simulink model "case7"  (R2024b)
settings: Solver=FixedStepAuto  StartTime=0  StopTime=1  FixedStep=1e-7  RelTol=1e-3
values from neighbouring files (symbols this model uses):
  SG_D_1_D = 0.01056    [IEEE9_case_parameters.m]    (also in case1_parameters.m; case2_parameters.m; case3_parameters.m; case4_parameters.m)
  SG_D_1_EnableSaturation = 0    [IEEE9_case_parameters.m]    (also in case1_parameters.m; case2_parameters.m; case3_parameters.m; case4_parameters.m)
  SG_D_1_f0 = 60    [IEEE9_case_parameters.m]    (also in case1_parameters.m; case2_parameters.m; case3_parameters.m; case4_parameters.m)
  SG_D_1_H = 7.5    [IEEE9_case_parameters.m]    (also in case1_parameters.m; case2_parameters.m; case3_parameters.m; case4_parameters.m)
  SG_D_1_K_A = 20    [IEEE9_case_parameters.m]    (also in case1_parameters.m; case2_parameters.m; case3_parameters.m; case4_parameters.m)
  SG_D_1_K_E = 1.000000e+1    (= 10)    [IEEE9_case_parameters.m]    (also in case1_parameters.m; case2_parameters.m; case3_parameters.m; case4_parameters.m)
  SG_D_1_K_F = 2.363    [IEEE9_case_parameters.m]    (also in case1_parameters.m; case2_parameters.m; case3_parameters.m; case4_parameters.m)
  SG_D_1_K_s = 0.5    [IEEE9_case_parameters.m]    (also in case1_parameters.m = 5; case2_parameters.m = 5; case3_parameters.m = 5; case4_parameters.m = 5)
  SG_D_1_R_a = 0.001088    [IEEE9_case_parameters.m]    (also in case1_parameters.m; case2_parameters.m; case3_parameters.m; case4_parameters.m)
  SG_D_1_S_A = 1    [IEEE9_case_parameters.m]    (also in case1_parameters.m; case2_parameters.m; case3_parameters.m; case4_parameters.m)
  SG_D_1_S_B = 0.103    [IEEE9_case_parameters.m]    (also in case1_parameters.m; case2_parameters.m; case3_parameters.m; case4_parameters.m)
  SG_D_1_S_N = 10.659857    [IEEE9_case_parameters.m]    (also in case1_parameters.m; case2_parameters.m; case3_parameters.m; case4_parameters.m)
  SG_D_1_SpeedPara = 200    [IEEE9_case_parameters.m]    (also in case1_parameters.m; case2_parameters.m; case3_parameters.m; case4_parameters.m)
  SG_D_1_T_0 = 0.720173    [IEEE9_case_parameters.m]    (also in case1_parameters.m = 0.755522; case2_parameters.m = 0.808931; case3_parameters.m = 0.869402; case4_parameters.m = 0.729316)
  SG_D_1_T_1 = 0.3    [IEEE9_case_parameters.m]    (also in case1_parameters.m; case2_parameters.m; case3_parameters.m; case4_parameters.m)
  SG_D_1_T_2 = 0.05    [IEEE9_case_parameters.m]    (also in case1_parameters.m; case2_parameters.m; case3_parameters.m; case4_parameters.m)
  SG_D_1_T_3 = 0.02    [IEEE9_case_parameters.m]    (also in case1_parameters.m; case2_parameters.m; case3_parameters.m; case4_parameters.m)
  SG_D_1_T_4 = 0.005    [IEEE9_case_parameters.m]    (also in case1_parameters.m; case2_parameters.m; case3_parameters.m; case4_parameters.m)
  SG_D_1_T_A = 0.02    [IEEE9_case_parameters.m]    (also in case1_parameters.m; case2_parameters.m; case3_parameters.m; case4_parameters.m)
  SG_D_1_T_dd = 8.000000e+0    (= 8)    [IEEE9_case_parameters.m]    (also in case1_parameters.m; case2_parameters.m; case3_parameters.m; case4_parameters.m)
  SG_D_1_T_ddd = 0.04    [IEEE9_case_parameters.m]    (also in case1_parameters.m; case2_parameters.m; case3_parameters.m; case4_parameters.m)
  SG_D_1_T_E = 0.314    [IEEE9_case_parameters.m]    (also in case1_parameters.m; case2_parameters.m; case3_parameters.m; case4_parameters.m)
  SG_D_1_T_F = 0.35    [IEEE9_case_parameters.m]    (also in case1_parameters.m; case2_parameters.m; case3_parameters.m; case4_parameters.m)
  SG_D_1_T_qd = 0.8    [IEEE9_case_parameters.m]    (also in case1_parameters.m; case2_parameters.m; case3_parameters.m; case4_parameters.m)
  SG_D_1_T_qdd = 0.02    [IEEE9_case_parameters.m]    (also in case1_parameters.m; case2_parameters.m; case3_parameters.m; case4_parameters.m)
  SG_D_1_T_speed = 0.1    [IEEE9_case_parameters.m]    (also in case1_parameters.m = 200; case2_parameters.m = 200; case3_parameters.m = 200; case4_parameters.m = 200)
  SG_D_1_T_w = 0.5    [IEEE9_case_parameters.m]    (also in case1_parameters.m; case2_parameters.m; case3_parameters.m; case4_parameters.m)
  SG_D_1_V_ref = 1.990276    [IEEE9_case_parameters.m]    (also in case1_parameters.m = 2.042296; case2_parameters.m = 2.051388; case3_parameters.m = 2.089584; case4_parameters.m = 2.01845)
  SG_D_1_w_ref = 376.991118    [IEEE9_case_parameters.m]    (also in case1_parameters.m; case2_parameters.m; case3_parameters.m; case4_parameters.m)
  SG_D_1_wb = 6.000000e+1    (= 60)    [IEEE9_case_parameters.m]    (also in case1_parameters.m; case2_parameters.m; case3_parameters.m; case4_parameters.m)
  SG_D_1_x_d = 1.9    [IEEE9_case_parameters.m]    (also in case1_parameters.m; case2_parameters.m; case3_parameters.m; case4_parameters.m)
  SG_D_1_x_dd = 0.302    [IEEE9_case_parameters.m]    (also in case1_parameters.m; case2_parameters.m; case3_parameters.m; case4_parameters.m)
  SG_D_1_x_ddd = 0.204    [IEEE9_case_parameters.m]    (also in case1_parameters.m; case2_parameters.m; case3_parameters.m; case4_parameters.m)
  SG_D_1_x_l = 0.05    [IEEE9_case_parameters.m]    (also in case1_parameters.m; case2_parameters.m; case3_parameters.m; case4_parameters.m)
  SG_D_1_x_q = 1.3    [IEEE9_case_parameters.m]    (also in case1_parameters.m; case2_parameters.m; case3_parameters.m; case4_parameters.m)
  SG_D_1_x_qd = 0.5    [IEEE9_case_parameters.m]    (also in case1_parameters.m; case2_parameters.m; case3_parameters.m; case4_parameters.m)
  SG_D_1_x_qdd = 0.3    [IEEE9_case_parameters.m]    (also in case1_parameters.m; case2_parameters.m; case3_parameters.m; case4_parameters.m)
  SG_D_2_D = 0.02    [IEEE9_case_parameters.m]    (also in case1_parameters.m; case2_parameters.m; case3_parameters.m; case4_parameters.m)
  SG_D_2_EnableSaturation = 0    [IEEE9_case_parameters.m]    (also in case1_parameters.m; case2_parameters.m; case3_parameters.m; case4_parameters.m)
  SG_D_2_f0 = 60    [IEEE9_case_parameters.m]    (also in case1_parameters.m; case2_parameters.m; case3_parameters.m; case4_parameters.m)
  SG_D_2_H = 8.000000e+0    (= 8)    [IEEE9_case_parameters.m]    (also in case1_parameters.m; case2_parameters.m; case3_parameters.m; case4_parameters.m)
  SG_D_2_K_A = 20    [IEEE9_case_parameters.m]    (also in case1_parameters.m; case2_parameters.m; case3_parameters.m; case4_parameters.m)
  SG_D_2_K_E = 1.000000e+1    (= 10)    [IEEE9_case_parameters.m]    (also in case1_parameters.m; case2_parameters.m; case3_parameters.m; case4_parameters.m)
  SG_D_2_K_F = 2.363    [IEEE9_case_parameters.m]    (also in case1_parameters.m; case2_parameters.m; case3_parameters.m; case4_parameters.m)
  SG_D_2_K_s = 0.5    [IEEE9_case_parameters.m]    (also in case1_parameters.m = 4; case2_parameters.m = 4; case3_parameters.m = 4; case4_parameters.m = 4)
  SG_D_2_R_a = 0.001088    [IEEE9_case_parameters.m]    (also in case1_parameters.m; case2_parameters.m; case3_parameters.m; case4_parameters.m)
  SG_D_2_S_A = 1    [IEEE9_case_parameters.m]    (also in case1_parameters.m; case2_parameters.m; case3_parameters.m; case4_parameters.m)
  SG_D_2_S_B = 0.103    [IEEE9_case_parameters.m]    (also in case1_parameters.m; case2_parameters.m; case3_parameters.m; case4_parameters.m)
  SG_D_2_S_N = 10.659857    [IEEE9_case_parameters.m]    (also in case1_parameters.m; case2_parameters.m; case3_parameters.m; case4_parameters.m)
  SG_D_2_SpeedPara = 200    [IEEE9_case_parameters.m]    (also in case1_parameters.m; case2_parameters.m; case3_parameters.m; case4_parameters.m)
  SG_D_2_T_0 = 1.632913    [IEEE9_case_parameters.m]    (also in case1_parameters.m = 1.632925; case2_parameters.m = 1.632915; case3_parameters.m = 1.632914; case4_parameters.m = 1.632927)
  SG_D_2_T_1 = 0.2    [IEEE9_case_parameters.m]    (also in case1_parameters.m; case2_parameters.m; case3_parameters.m; case4_parameters.m)
  SG_D_2_T_2 = 0.05    [IEEE9_case_parameters.m]    (also in case1_parameters.m; case2_parameters.m; case3_parameters.m; case4_parameters.m)
  SG_D_2_T_3 = 0.02    [IEEE9_case_parameters.m]    (also in case1_parameters.m; case2_parameters.m; case3_parameters.m; case4_parameters.m)
  SG_D_2_T_4 = 0.005    [IEEE9_case_parameters.m]    (also in case1_parameters.m; case2_parameters.m; case3_parameters.m; case4_parameters.m)
  SG_D_2_T_A = 0.02    [IEEE9_case_parameters.m]    (also in case1_parameters.m; case2_parameters.m; case3_parameters.m; case4_parameters.m)
  SG_D_2_T_dd = 7.9    [IEEE9_case_parameters.m]    (also in case1_parameters.m; case2_parameters.m; case3_parameters.m; case4_parameters.m)
  SG_D_2_T_ddd = 0.04    [IEEE9_case_parameters.m]    (also in case1_parameters.m; case2_parameters.m; case3_parameters.m; case4_parameters.m)
  SG_D_2_T_E = 0.314    [IEEE9_case_parameters.m]    (also in case1_parameters.m; case2_parameters.m; case3_parameters.m; case4_parameters.m)
  SG_D_2_T_F = 0.35    [IEEE9_case_parameters.m]    (also in case1_parameters.m; case2_parameters.m; case3_parameters.m; case4_parameters.m)
  SG_D_2_T_qd = 0.8    [IEEE9_case_parameters.m]    (also in case1_parameters.m; case2_parameters.m; case3_parameters.m; case4_parameters.m)
  SG_D_2_T_qdd = 0.015    [IEEE9_case_parameters.m]    (also in case1_parameters.m; case2_parameters.m; case3_parameters.m; case4_parameters.m)
  SG_D_2_T_speed = 0.1    [IEEE9_case_parameters.m]    (also in case1_parameters.m = 150; case2_parameters.m = 150; case3_parameters.m = 150; case4_parameters.m = 150)
  SG_D_2_T_w = 0.35    [IEEE9_case_parameters.m]    (also in case1_parameters.m; case2_parameters.m; case3_parameters.m; case4_parameters.m)
  SG_D_2_V_ref = 2.58547    [IEEE9_case_parameters.m]    (also in case1_parameters.m = 2.597896; case2_parameters.m = 2.587136; case3_parameters.m = 2.586042; case4_parameters.m = 2.599679)
  SG_D_2_w_ref = 376.991118    [IEEE9_case_parameters.m]    (also in case1_parameters.m; case2_parameters.m; case3_parameters.m; case4_parameters.m)
  SG_D_2_wb = 6.000000e+1    (= 60)    [IEEE9_case_parameters.m]    (also in case1_parameters.m; case2_parameters.m; case3_parameters.m; case4_parameters.m)
  SG_D_2_x_d = 1.8    [IEEE9_case_parameters.m]    (also in case1_parameters.m; case2_parameters.m; case3_parameters.m; case4_parameters.m)
  SG_D_2_x_dd = 0.302    [IEEE9_case_parameters.m]    (also in case1_parameters.m; case2_parameters.m; case3_parameters.m; case4_parameters.m)
  SG_D_2_x_ddd = 0.204    [IEEE9_case_parameters.m]    (also in case1_parameters.m; case2_parameters.m; case3_parameters.m; case4_parameters.m)
  SG_D_2_x_l = 0.05    [IEEE9_case_parameters.m]    (also in case1_parameters.m; case2_parameters.m; case3_parameters.m; case4_parameters.m)
  SG_D_2_x_q = 1.25    [IEEE9_case_parameters.m]    (also in case1_parameters.m; case2_parameters.m; case3_parameters.m; case4_parameters.m)
  SG_D_2_x_qd = 0.5    [IEEE9_case_parameters.m]    (also in case1_parameters.m; case2_parameters.m; case3_parameters.m; case4_parameters.m)
  SG_D_2_x_qdd = 0.3    [IEEE9_case_parameters.m]    (also in case1_parameters.m; case2_parameters.m; case3_parameters.m; case4_parameters.m)
  SG_D_3_D = 0.02    [IEEE9_case_parameters.m]    (also in case1_parameters.m; case2_parameters.m; case3_parameters.m; case4_parameters.m)
  SG_D_3_EnableSaturation = 0    [IEEE9_case_parameters.m]    (also in case1_parameters.m; case2_parameters.m; case3_parameters.m; case4_parameters.m)
  SG_D_3_f0 = 60    [IEEE9_case_parameters.m]    (also in case1_parameters.m; case2_parameters.m; case3_parameters.m; case4_parameters.m)
  SG_D_3_H = 7.7    [IEEE9_case_parameters.m]    (also in case1_parameters.m; case2_parameters.m; case3_parameters.m; case4_parameters.m)
  SG_D_3_K_A = 20    [IEEE9_case_parameters.m]    (also in case1_parameters.m; case2_parameters.m; case3_parameters.m; case4_parameters.m)
  SG_D_3_K_E = 1.000000e+1    (= 10)    [IEEE9_case_parameters.m]    (also in case1_parameters.m; case2_parameters.m; case3_parameters.m; case4_parameters.m)
  SG_D_3_K_F = 2.363    [IEEE9_case_parameters.m]    (also in case1_parameters.m; case2_parameters.m; case3_parameters.m; case4_parameters.m)
  SG_D_3_K_s = 0.2    [IEEE9_case_parameters.m]    (also in case1_parameters.m = 2; case2_parameters.m = 2; case3_parameters.m = 2; case4_parameters.m = 2)
  SG_D_3_R_a = 0.001088    [IEEE9_case_parameters.m]    (also in case1_parameters.m; case2_parameters.m; case3_parameters.m; case4_parameters.m)
  SG_D_3_S_A = 1    [IEEE9_case_parameters.m]    (also in case1_parameters.m; case2_parameters.m; case3_parameters.m; case4_parameters.m)
  SG_D_3_S_B = 0.103    [IEEE9_case_parameters.m]    (also in case1_parameters.m; case2_parameters.m; case3_parameters.m; case4_parameters.m)
  SG_D_3_S_N = 10.659857    [IEEE9_case_parameters.m]    (also in case1_parameters.m; case2_parameters.m; case3_parameters.m; case4_parameters.m)
  SG_D_3_SpeedPara = 200    [IEEE9_case_parameters.m]    (also in case1_parameters.m; case2_parameters.m; case3_parameters.m; case4_parameters.m)
  SG_D_3_T_0 = 0.850788    [IEEE9_case_parameters.m]    (also in case1_parameters.m = 0.850786; case2_parameters.m = 0.850787; case3_parameters.m; case4_parameters.m = 0.850786)
  SG_D_3_T_1 = 0.2    [IEEE9_case_parameters.m]    (also in case1_parameters.m; case2_parameters.m; case3_parameters.m; case4_parameters.m)
  SG_D_3_T_2 = 0.05    [IEEE9_case_parameters.m]    (also in case1_parameters.m; case2_parameters.m; case3_parameters.m; case4_parameters.m)
  SG_D_3_T_3 = 0.02    [IEEE9_case_parameters.m]    (also in case1_parameters.m; case2_parameters.m; case3_parameters.m; case4_parameters.m)
  SG_D_3_T_4 = 0.005    [IEEE9_case_parameters.m]    (also in case1_parameters.m; case2_parameters.m; case3_parameters.m; case4_parameters.m)
  SG_D_3_T_A = 0.02    [IEEE9_case_parameters.m]    (also in case1_parameters.m; case2_parameters.m; case3_parameters.m; case4_parameters.m)
  SG_D_3_T_dd = 8.1    [IEEE9_case_parameters.m]    (also in case1_parameters.m; case2_parameters.m; case3_parameters.m; case4_parameters.m)
  SG_D_3_T_ddd = 0.04    [IEEE9_case_parameters.m]    (also in case1_parameters.m; case2_parameters.m; case3_parameters.m; case4_parameters.m)
  SG_D_3_T_E = 0.314    [IEEE9_case_parameters.m]    (also in case1_parameters.m; case2_parameters.m; case3_parameters.m; case4_parameters.m)
  SG_D_3_T_F = 0.35    [IEEE9_case_parameters.m]    (also in case1_parameters.m; case2_parameters.m; case3_parameters.m; case4_parameters.m)
  SG_D_3_T_qd = 0.8    [IEEE9_case_parameters.m]    (also in case1_parameters.m; case2_parameters.m; case3_parameters.m; case4_parameters.m)
  SG_D_3_T_qdd = 0.015    [IEEE9_case_parameters.m]    (also in case1_parameters.m; case2_parameters.m; case3_parameters.m; case4_parameters.m)
  SG_D_3_T_speed = 0.1    [IEEE9_case_parameters.m]    (also in case1_parameters.m = 180; case2_parameters.m = 180; case3_parameters.m = 180; case4_parameters.m = 180)
  SG_D_3_T_w = 0.4    [IEEE9_case_parameters.m]    (also in case1_parameters.m; case2_parameters.m; case3_parameters.m; case4_parameters.m)
  SG_D_3_V_ref = 1.892727    [IEEE9_case_parameters.m]    (also in case1_parameters.m = 1.906439; case2_parameters.m = 1.895535; case3_parameters.m = 1.892105; case4_parameters.m = 1.906598)
  SG_D_3_w_ref = 376.991118    [IEEE9_case_parameters.m]    (also in case1_parameters.m; case2_parameters.m; case3_parameters.m; case4_parameters.m)
  SG_D_3_wb = 6.000000e+1    (= 60)    [IEEE9_case_parameters.m]    (also in case1_parameters.m; case2_parameters.m; case3_parameters.m; case4_parameters.m)
  SG_D_3_x_d = 1.85    [IEEE9_case_parameters.m]    (also in case1_parameters.m; case2_parameters.m; case3_parameters.m; case4_parameters.m)
  SG_D_3_x_dd = 0.302    [IEEE9_case_parameters.m]    (also in case1_parameters.m; case2_parameters.m; case3_parameters.m; case4_parameters.m)
  SG_D_3_x_ddd = 0.204    [IEEE9_case_parameters.m]    (also in case1_parameters.m; case2_parameters.m; case3_parameters.m; case4_parameters.m)
  SG_D_3_x_l = 0.05    [IEEE9_case_parameters.m]    (also in case1_parameters.m; case2_parameters.m; case3_parameters.m; case4_parameters.m)
  SG_D_3_x_q = 1.2    [IEEE9_case_parameters.m]    (also in case1_parameters.m; case2_parameters.m; case3_parameters.m; case4_parameters.m)
  SG_D_3_x_qd = 0.5    [IEEE9_case_parameters.m]    (also in case1_parameters.m; case2_parameters.m; case3_parameters.m; case4_parameters.m)
  SG_D_3_x_qdd = 0.3    [IEEE9_case_parameters.m]    (also in case1_parameters.m; case2_parameters.m; case3_parameters.m; case4_parameters.m)
(part 6 of 12)

== system case7/SG_D_1/d_psi_kq_SG_D_1_block ==
  note: d_psi_kq_SG_D_1 in case7
      | $-\frac{\psi _{\mathrm{gq},\mathrm{SG},D,1}+\psi _{\mathrm{kq},\mathrm{SG},D,1}+\frac{\left(x_{l}-x_{\mathrm{qd}}\right)\,\left(\psi _{q,\mathrm{SG},D,1}+\frac{\psi _{\mathrm{gq},\mathrm{SG},D,1}\,\left(x_{l}-x_{\mathrm{qdd}}\right)}{x_{l}-x_{\mathrm{qd}}}+\frac{\psi _{\mathrm{kq},\mathrm{SG},D,1}\,\left(x_{\mathrm{qd}}-x_{\mathrm{qdd}}\right)}{x_{l}-x_{\mathrm{qd}}}\right)}{x_{\mathrm{qdd}}}}{T_{\mathrm{qdd}}}$
      | Automatically generated on 2025-10-31 19:23:24 .
  State_psi_gq_SG_D_1_141c0 : Inport
  State_psi_kq_SG_D_1_73ccc : Inport  Port=2
  State_psi_gq_SG_D_1_32f50 : Inport  Port=3
  State_psi_kq_SG_D_1_9c021 : Inport  Port=4
  State_psi_q_SG_D_1_95dfc : Inport  Port=5
  Add_4d238 : Sum
  Add_52c21 : Sum
  Add_5b3bd : Sum
  Add_78e01 : Sum
  Add_7e5bc : Sum
  Add_abf74 : Sum
  Constant_-1_7f4f9 : Constant  Value=-1
  Constant_-1_8033d : Constant  Value=-1
  Constant_-1_939f1 : Constant  Value=-1
  Constant_-1_ca431 : Constant  Value=-1
  Constant_-1_cc594 : Constant  Value=-1
  Constant_T_qdd_ef478 : Constant  Value=T_qdd
  Constant_x_l_00713 : Constant  Value=x_l
  Constant_x_l_01d91 : Constant  Value=x_l
  Constant_x_l_4eb42 : Constant  Value=x_l
  Constant_x_l_702c1 : Constant  Value=x_l
  Constant_x_qd_06ea1 : Constant  Value=x_qd
  Constant_x_qd_55376 : Constant  Value=x_qd
  Constant_x_qd_bc9ff : Constant  Value=x_qd
  Constant_x_qd_cd86c : Constant  Value=x_qd
  Constant_x_qdd_04518 : Constant  Value=x_qdd
  Constant_x_qdd_b13f8 : Constant  Value=x_qdd
  Constant_x_qdd_e31b1 : Constant  Value=x_qdd
  Divide_172d7 : Product  Inputs=*/
  Divide_318ea : Product  Inputs=*/
  Divide_dd02d : Product  Inputs=*/
  Divide_ff5c9 : Product  Inputs=*/
  Product_49e9a : Product
  Product_575bc : Product
  Product_595ac : Product
  Product_801da : Product
  Product_92b80 : Product
  Product_9c9eb : Product
  Product_d5d1d : Product
  Product_e2544 : Product
  Subtract_41446 : Sum  Inputs=+-
  Subtract_9a187 : Sum  Inputs=+-
  Subtract_c7d32 : Sum  Inputs=+-
  Blockout_d_psi_kq_SG_D_1_55298 : Outport
  wires:
  Product_e2544/1 -> Add_5b3bd/1
  Constant_-1_cc594/1 -> Product_e2544/1
  Constant_x_l_01d91/1 -> Product_e2544/2
  Constant_x_qdd_b13f8/1 -> Add_5b3bd/2
  Constant_-1_8033d/1 -> Product_9c9eb/1
  Constant_x_qd_cd86c/1 -> Subtract_9a187/1
  Constant_x_qd_bc9ff/1 -> Add_7e5bc/2
  Constant_-1_939f1/1 -> Product_575bc/1
  Constant_x_l_4eb42/1 -> Product_9c9eb/2
  Constant_x_qdd_04518/1 -> Subtract_9a187/2
  Constant_x_qd_06ea1/1 -> Add_52c21/2
  Constant_x_l_00713/1 -> Product_575bc/2
  Subtract_41446/1 -> Add_78e01/1
  Product_801da/1 -> Subtract_41446/1
  State_psi_gq_SG_D_1_32f50/1 -> Product_92b80/1
  Add_5b3bd/1 -> Product_92b80/2
  Product_575bc/1 -> Add_4d238/1
  Constant_x_qd_55376/1 -> Add_4d238/2
  State_psi_kq_SG_D_1_9c021/1 -> Product_595ac/1
  Product_9c9eb/1 -> Add_52c21/1
  Subtract_9a187/1 -> Product_595ac/2
  Product_92b80/1 -> Divide_ff5c9/1
  Add_4d238/1 -> Divide_ff5c9/2
  Product_595ac/1 -> Divide_318ea/1
  Add_52c21/1 -> Divide_318ea/2
  Constant_-1_7f4f9/1 -> Product_d5d1d/1
  Constant_x_l_702c1/1 -> Product_d5d1d/2
  Divide_ff5c9/1 -> Subtract_c7d32/1
  Divide_318ea/1 -> Subtract_c7d32/2
  Product_d5d1d/1 -> Add_7e5bc/1
  Add_abf74/1 -> Product_49e9a/2
  Subtract_c7d32/1 -> Add_abf74/1
  State_psi_q_SG_D_1_95dfc/1 -> Add_abf74/2
  Constant_-1_ca431/1 -> Product_801da/1
  State_psi_gq_SG_D_1_141c0/1 -> Product_801da/2
  Divide_172d7/1 -> Add_78e01/2
  Product_49e9a/1 -> Divide_172d7/1
  Add_7e5bc/1 -> Product_49e9a/1
  State_psi_kq_SG_D_1_73ccc/1 -> Subtract_41446/2
  Constant_x_qdd_e31b1/1 -> Divide_172d7/2
  Add_78e01/1 -> Divide_dd02d/1
  Constant_T_qdd_ef478/1 -> Divide_dd02d/2
  Divide_dd02d/1 -> Blockout_d_psi_kq_SG_D_1_55298/1

== system case7/SG_D_1/d_psi_q_SG_D_1_block ==
  note: d_psi_q_SG_D_1 in case7
      | $2\,\pi \,f_{0}\,\left(v_{d,\mathrm{SG},D,1}\,\cos\left(\theta _{\mathrm{SG},D,1}\right)+v_{q,\mathrm{SG},D,1}\,\sin\left(\theta _{\mathrm{SG},D,1}\right)-\frac{R_{a}\,\left(\psi _{q,\mathrm{SG},D,1}+\frac{\psi _{\mathrm{gq},\mathrm{SG},D,1}\,\left(x_{l}-x_{\mathrm{qdd}}\right)}{x_{l}-x_{\mathrm{qd}}}+\frac{\psi _{\mathrm{kq},\mathrm{SG},D,1}\,\left(x_{\mathrm{qd}}-x_{\mathrm{qdd}}\right)}{x_{l}-x_{\mathrm{qd}}}\right)}{x_{\mathrm{qdd}}}-\frac{\psi _{d,\mathrm{SG},D,1}\,w_{\mathrm{SG},D,1}}{2\,f_{0}\,\pi }\right)$
      | Automatically generated on 2025-10-31 19:23:07 .
  State_psi_gq_SG_D_1_4f3e1 : Inport
  State_psi_kq_SG_D_1_8ab4d : Inport  Port=2
  State_psi_q_SG_D_1_9b7b7 : Inport  Port=3
  Input_v_d_SG_D_1_5bf66 : Inport  Port=4
  State_theta_SG_D_1_45d91 : Inport  Port=5
  Input_v_q_SG_D_1_520ac : Inport  Port=6
  State_theta_SG_D_1_c7f9c : Inport  Port=7
  State_psi_d_SG_D_1_d17e6 : Inport  Port=8
  State_w_SG_D_1_b7eed : Inport  Port=9
  Add_243db : Sum
  Add_43c61 : Sum
  Add_a9329 : Sum
  Add_e3412 : Sum
  Add_f2e06 : Sum
  Constant_-1_319d6 : Constant  Value=-1
  Constant_-1_3e2ef : Constant  Value=-1
  Constant_-1_43b5b : Constant  Value=-1
  Constant_-2.0_d2834 : Constant  Value=-2.0
  Constant_2.0_6844f : Constant  Value=2.0
  Constant_R_a_25f1c : Constant  Value=R_a
  Constant_f0_e7b9b : Constant  Value=f0
  Constant_f0_edef6 : Constant  Value=f0
  Constant_pi_68b7d : Constant  Value=pi
  Constant_pi_ccff0 : Constant  Value=pi
  Constant_x_l_9a800 : Constant  Value=x_l
  Constant_x_l_c28ae : Constant  Value=x_l
  Constant_x_l_f0117 : Constant  Value=x_l
  Constant_x_qd_683b7 : Constant  Value=x_qd
  Constant_x_qd_af3ac : Constant  Value=x_qd
  Constant_x_qd_e0e5a : Constant  Value=x_qd
  Constant_x_qdd_0e5be : Constant  Value=x_qdd
  Constant_x_qdd_ca234 : Constant  Value=x_qdd
  Constant_x_qdd_e9210 : Constant  Value=x_qdd
  Divide_0e09a : Product  Inputs=*/
  Divide_18e9c : Product  Inputs=*/
  Divide_2196d : Product  Inputs=*/
  Divide_8c0c5 : Product  Inputs=*/
  MathFunc_cos_7ee3d : Trigonometry  Operator=cos
  MathFunc_sin_228e5 : Trigonometry
  Product_0c91d : Product
  Product_373f1 : Product
  Product_40236 : Product
  Product_41ef0 : Product
  Product_47c5e : Product
  Product_51a0c : Product
  Product_5cef1 : Product
  Product_67a0a : Product
  Product_78b72 : Product
  Product_7b854 : Product
  Product_8d118 : Product
  Product_95aa7 : Product
  Product_aa900 : Product
  Product_ff687 : Product
  Subtract_0ff74 : Sum  Inputs=+-
  Subtract_1a25f : Sum  Inputs=+-
  Subtract_c693d : Sum  Inputs=+-
  Subtract_f016c : Sum  Inputs=+-
  Blockout_d_psi_q_SG_D_1_cd2a8 : Outport
  wires:
  Divide_0e09a/1 -> Subtract_f016c/1
  Product_373f1/1 -> Add_f2e06/1
  Constant_x_l_c28ae/1 -> Product_373f1/2
  Constant_-1_3e2ef/1 -> Product_373f1/1
  Constant_x_qdd_ca234/1 -> Add_f2e06/2
  Constant_x_l_f0117/1 -> Product_67a0a/2
  Constant_-1_319d6/1 -> Product_67a0a/1
  Constant_x_l_9a800/1 -> Product_95aa7/2
  Constant_x_qdd_0e5be/1 -> Subtract_c693d/2
  State_psi_kq_SG_D_1_8ab4d/1 -> Product_51a0c/1
  Constant_-1_43b5b/1 -> Product_95aa7/1
  Constant_x_qd_e0e5a/1 -> Subtract_c693d/1
  State_psi_gq_SG_D_1_4f3e1/1 -> Product_aa900/1
  Product_47c5e/1 -> Blockout_d_psi_q_SG_D_1_cd2a8/1
  Subtract_f016c/1 -> Add_e3412/1
  Product_aa900/1 -> Divide_0e09a/1
  Add_f2e06/1 -> Product_aa900/2
  Divide_8c0c5/1 -> Subtract_f016c/2
  Product_67a0a/1 -> Add_43c61/1
  Constant_x_qd_af3ac/1 -> Add_43c61/2
  Constant_-2.0_d2834/1 -> Product_40236/1
  Product_51a0c/1 -> Divide_8c0c5/1
  Product_95aa7/1 -> Add_a9329/1
  Subtract_c693d/1 -> Product_51a0c/2
  Constant_x_qd_683b7/1 -> Add_a9329/2
  Add_43c61/1 -> Divide_0e09a/2
  Add_a9329/1 -> Divide_8c0c5/2
  Constant_f0_edef6/1 -> Product_5cef1/2
  State_psi_q_SG_D_1_9b7b7/1 -> Add_e3412/2
  Product_7b854/1 -> Product_ff687/1
  Constant_R_a_25f1c/1 -> Product_0c91d/1
  Product_ff687/1 -> Divide_18e9c/2
  Product_0c91d/1 -> Divide_2196d/1
  Add_e3412/1 -> Product_0c91d/2
  State_theta_SG_D_1_45d91/1 -> MathFunc_cos_7ee3d/1
  Input_v_d_SG_D_1_5bf66/1 -> Product_41ef0/1
  Constant_x_qdd_e9210/1 -> Divide_2196d/2
  MathFunc_cos_7ee3d/1 -> Product_41ef0/2
  State_theta_SG_D_1_c7f9c/1 -> MathFunc_sin_228e5/1
  Divide_2196d/1 -> Subtract_1a25f/1
  Constant_2.0_6844f/1 -> Product_7b854/1
  State_w_SG_D_1_b7eed/1 -> Product_78b72/2
  Constant_pi_68b7d/1 -> Product_7b854/2
  Subtract_0ff74/1 -> Add_243db/1
  Product_41ef0/1 -> Subtract_1a25f/2
  Divide_18e9c/1 -> Add_243db/2
  Input_v_q_SG_D_1_520ac/1 -> Product_8d118/1
  MathFunc_sin_228e5/1 -> Product_8d118/2
  Product_8d118/1 -> Subtract_0ff74/2
  State_psi_d_SG_D_1_d17e6/1 -> Product_78b72/1
  Constant_f0_e7b9b/1 -> Product_ff687/2
  Constant_pi_ccff0/1 -> Product_40236/2
  Subtract_1a25f/1 -> Subtract_0ff74/1
  Product_78b72/1 -> Divide_18e9c/1
  Product_40236/1 -> Product_5cef1/1
  Product_5cef1/1 -> Product_47c5e/1
  Add_243db/1 -> Product_47c5e/2

== system case7/SG_D_1/d_theta_SG_D_1_block ==
  note: d_theta_SG_D_1 in case7
      | $w_{\mathrm{SG},D,1}-2\,\pi \,f_{0}$
      | Automatically generated on 2025-10-31 19:23:31 .
  State_w_SG_D_1_8cf49 : Inport
  Add_3ec9b : Sum
  Constant_-2.0_16d25 : Constant  Value=-2.0
  Constant_f0_fa8b8 : Constant  Value=f0
  Constant_pi_3da35 : Constant  Value=pi
  Product_154ca : Product
  Product_7fb81 : Product
  Blockout_d_theta_SG_D_1_2a112 : Outport
  wires:
  State_w_SG_D_1_8cf49/1 -> Add_3ec9b/2
  Constant_-2.0_16d25/1 -> Product_7fb81/1
  Constant_f0_fa8b8/1 -> Product_154ca/2
  Constant_pi_3da35/1 -> Product_7fb81/2
  Product_154ca/1 -> Add_3ec9b/1
  Product_7fb81/1 -> Product_154ca/1
  Add_3ec9b/1 -> Blockout_d_theta_SG_D_1_2a112/1

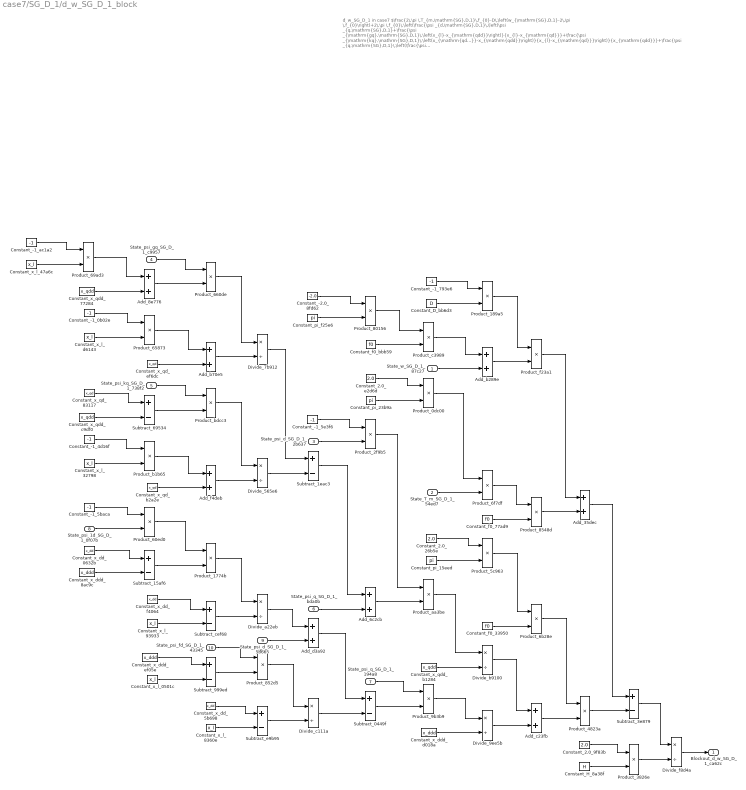
== system case7/SG_D_1/d_w_SG_D_1_block ==
  note: d_w_SG_D_1 in case7
      | $\frac{2\,\pi \,T_{m,\mathrm{SG},D,1}\,f_{0}-D\,\left(w_{\mathrm{SG},D,1}-2\,\pi \,f_{0}\right)+2\,\pi \,f_{0}\,\left(\frac{\psi _{d,\mathrm{SG},D,1}\,\left(\psi _{q,\mathrm{SG},D,1}+\frac{\psi _{\mathrm{gq},\mathrm{SG},D,1}\,\left(x_{l}-x_{\mathrm{qdd}}\right)}{x_{l}-x_{\mathrm{qd}}}+\frac{\psi _{\mathrm{kq},\mathrm{SG},D,1}\,\left(x_{\mathrm{qd}}-x_{\mathrm{qdd}}\right)}{x_{l}-x_{\mathrm{qd}}}\right)}{x_{\mathrm{qdd}}}+\frac{\psi _{q,\mathrm{SG},D,1}\,\left(\frac{\psi _{\mathrm{1d},\mathrm{SG},D,1}\,\left(x_{\mathrm{dd}}-x_{\mathrm{ddd}}\right)}{x_{\mathrm{dd}}-x_{l}}-\psi _{d,\mathrm{SG},D,1}+\frac{\psi _{\mathrm{fd},\mathrm{SG},D,1}\,\left(x_{\mathrm{ddd}}-x_{l}\right)}{x_{\mathrm{dd}}-x_{l}}\right)}{x_{\mathrm{ddd}}}\right)}{2\,H}$
      | Automatically generated on 2025-10-31 19:23:30 .
  State_w_SG_D_1_87c27 : Inport
  State_T_m_SG_D_1_54ed7 : Inport  Port=2
  State_psi_d_SG_D_1_2b637 : Inport  Port=3
  State_psi_gq_SG_D_1_c9957 : Inport  Port=4
  State_psi_kq_SG_D_1_738f2 : Inport  Port=5
  State_psi_q_SG_D_1_bda0b : Inport  Port=6
  State_psi_q_SG_D_1_194a8 : Inport  Port=7
  State_psi_1d_SG_D_1_0f07b : Inport  Port=8
  State_psi_d_SG_D_1_5b665 : Inport  Port=9
  State_psi_fd_SG_D_1_43345 : Inport  Port=10
  Add_35dec : Sum
  Add_6c2cb : Sum
  Add_8e776 : Sum
  Add_b289e : Sum
  Add_b70e5 : Sum
  Add_c23fb : Sum
  Add_d3a92 : Sum
  Add_f4deb : Sum
  Constant_-1_0b02e : Constant  Value=-1
  Constant_-1_4d16f : Constant  Value=-1
  Constant_-1_5baca : Constant  Value=-1
  Constant_-1_5e3f6 : Constant  Value=-1
  Constant_-1_793e6 : Constant  Value=-1
  Constant_-1_ac1a2 : Constant  Value=-1
  Constant_-2.0_8fd62 : Constant  Value=-2.0
  Constant_2.0_26b5e : Constant  Value=2.0
  Constant_2.0_9f83b : Constant  Value=2.0
  Constant_2.0_e2d6d : Constant  Value=2.0
  Constant_D_bb6d3 : Constant  Value=D
  Constant_H_8a38f : Constant  Value=H
  Constant_f0_33950 : Constant  Value=f0
  Constant_f0_77ad9 : Constant  Value=f0
  Constant_f0_bbb59 : Constant  Value=f0
  Constant_pi_15eed : Constant  Value=pi
  Constant_pi_23b9a : Constant  Value=pi
  Constant_pi_f25e6 : Constant  Value=pi
  Constant_x_dd_0632b : Constant  Value=x_dd
  Constant_x_dd_5b698 : Constant  Value=x_dd
  Constant_x_dd_f4064 : Constant  Value=x_dd
  Constant_x_ddd_8ac9c : Constant  Value=x_ddd
  Constant_x_ddd_d018a : Constant  Value=x_ddd
  Constant_x_ddd_ef05e : Constant  Value=x_ddd
  Constant_x_l_0501c : Constant  Value=x_l
  Constant_x_l_32798 : Constant  Value=x_l
  Constant_x_l_47a6c : Constant  Value=x_l
  Constant_x_l_8360e : Constant  Value=x_l
  Constant_x_l_93933 : Constant  Value=x_l
  Constant_x_l_d6143 : Constant  Value=x_l
  Constant_x_qd_83117 : Constant  Value=x_qd
  Constant_x_qd_b2a2e : Constant  Value=x_qd
  Constant_x_qd_ef6dc : Constant  Value=x_qd
  Constant_x_qdd_77284 : Constant  Value=x_qdd
  Constant_x_qdd_b1284 : Constant  Value=x_qdd
  Constant_x_qdd_c9df0 : Constant  Value=x_qdd
  Divide_565e6 : Product  Inputs=*/
  Divide_7b912 : Product  Inputs=*/
  Divide_9ee5b : Product  Inputs=*/
  Divide_a22eb : Product  Inputs=*/
  Divide_b9100 : Product  Inputs=*/
  Divide_c111a : Product  Inputs=*/
  Divide_f8d4a : Product  Inputs=*/
  Product_0dc00 : Product
  Product_1774b : Product
  Product_189a5 : Product
  Product_2f9b5 : Product
  Product_3826e : Product
  Product_4823a : Product
  Product_5c963 : Product
  Product_60ed0 : Product
  Product_65873 : Product
  Product_660de : Product
  Product_69ad3 : Product
  Product_6b28e : Product
  Product_6f7df : Product
  Product_80156 : Product
  Product_852d5 : Product
  Product_8548d : Product
  Product_9b3b9 : Product
  Product_aa3be : Product
  Product_b1b65 : Product
  Product_bdcc3 : Product
  Product_c3989 : Product
  Product_f23a1 : Product
  Subtract_0449f : Sum  Inputs=+-
  Subtract_15af6 : Sum  Inputs=+-
  Subtract_1eac3 : Sum  Inputs=+-
  Subtract_3e879 : Sum  Inputs=+-
  Subtract_69534 : Sum  Inputs=+-
  Subtract_999ed : Sum  Inputs=+-
  Subtract_cef68 : Sum  Inputs=+-
  Subtract_e9b95 : Sum  Inputs=+-
  Blockout_d_w_SG_D_1_ca62c : Outport
  wires:
  Product_c3989/1 -> Add_b289e/1
  Constant_-1_ac1a2/1 -> Product_69ad3/1
  Constant_pi_23b9a/1 -> Product_0dc00/2
  Constant_x_qdd_77284/1 -> Add_8e776/2
  Constant_x_l_47a6c/1 -> Product_69ad3/2
  Product_69ad3/1 -> Add_8e776/1
  Constant_x_qd_83117/1 -> Subtract_69534/1
  Constant_-1_0b02e/1 -> Product_65873/1
  Product_80156/1 -> Product_c3989/1
  Constant_x_qdd_c9df0/1 -> Subtract_69534/2
  State_psi_q_SG_D_1_194a8/1 -> Product_9b3b9/1
  Constant_x_l_d6143/1 -> Product_65873/2
  Constant_-1_4d16f/1 -> Product_b1b65/1
  Constant_x_l_32798/1 -> Product_b1b65/2
  Constant_-1_5baca/1 -> Product_60ed0/1
  Product_65873/1 -> Add_b70e5/1
  State_psi_1d_SG_D_1_0f07b/1 -> Product_60ed0/2
  Constant_x_dd_0632b/1 -> Subtract_15af6/1
  Subtract_69534/1 -> Product_bdcc3/2
  Constant_x_ddd_8ac9c/1 -> Subtract_15af6/2
  State_psi_gq_SG_D_1_c9957/1 -> Product_660de/1
  Product_2f9b5/1 -> Product_aa3be/1
  Add_8e776/1 -> Product_660de/2
  Constant_x_qd_ef6dc/1 -> Add_b70e5/2
  State_psi_kq_SG_D_1_738f2/1 -> Product_bdcc3/1
  Constant_f0_bbb59/1 -> Product_c3989/2
  Product_b1b65/1 -> Add_f4deb/1
  Constant_x_dd_f4064/1 -> Subtract_cef68/1
  Constant_x_qd_b2a2e/1 -> Add_f4deb/2
  Product_60ed0/1 -> Product_1774b/1
  Subtract_15af6/1 -> Product_1774b/2
  Constant_x_l_93933/1 -> Subtract_cef68/2
  Constant_x_ddd_ef05e/1 -> Subtract_999ed/1
  Constant_x_l_0501c/1 -> Subtract_999ed/2
  State_w_SG_D_1_87c27/1 -> Add_b289e/2
  Divide_b9100/1 -> Add_c23fb/1
  Constant_-1_793e6/1 -> Product_189a5/1
  Product_660de/1 -> Divide_7b912/1
  Add_b289e/1 -> Product_f23a1/2
  Divide_7b912/1 -> Subtract_1eac3/1
  Add_b70e5/1 -> Divide_7b912/2
  Constant_pi_f25e6/1 -> Product_80156/2
  Product_bdcc3/1 -> Divide_565e6/1
  Add_f4deb/1 -> Divide_565e6/2
  Product_1774b/1 -> Divide_a22eb/1
  Divide_a22eb/1 -> Add_d3a92/1
  Subtract_cef68/1 -> Divide_a22eb/2
  State_psi_fd_SG_D_1_43345/1 -> Product_852d5/1
  Subtract_999ed/1 -> Product_852d5/2
  Constant_x_dd_5b698/1 -> Subtract_e9b95/1
  Constant_x_l_8360e/1 -> Subtract_e9b95/2
  Divide_565e6/1 -> Subtract_1eac3/2
  Constant_2.0_e2d6d/1 -> Product_0dc00/1
  State_psi_d_SG_D_1_5b665/1 -> Add_d3a92/2
  Product_852d5/1 -> Divide_c111a/1
  Subtract_e9b95/1 -> Divide_c111a/2
  Constant_-2.0_8fd62/1 -> Product_80156/1
  Constant_-1_5e3f6/1 -> Product_2f9b5/1
  State_psi_d_SG_D_1_2b637/1 -> Product_2f9b5/2
  Subtract_1eac3/1 -> Add_6c2cb/1
  Subtract_0449f/1 -> Product_9b3b9/2
  State_psi_q_SG_D_1_bda0b/1 -> Add_6c2cb/2
  Add_d3a92/1 -> Subtract_0449f/1
  Divide_c111a/1 -> Subtract_0449f/2
  Add_6c2cb/1 -> Product_aa3be/2
  Constant_D_bb6d3/1 -> Product_189a5/2
  Product_0dc00/1 -> Product_6f7df/1
  State_T_m_SG_D_1_54ed7/1 -> Product_6f7df/2
  Constant_2.0_26b5e/1 -> Product_5c963/1
  Constant_pi_15eed/1 -> Product_5c963/2
  Product_aa3be/1 -> Divide_b9100/1
  Constant_x_qdd_b1284/1 -> Divide_b9100/2
  Product_9b3b9/1 -> Divide_9ee5b/1
  Constant_x_ddd_d018a/1 -> Divide_9ee5b/2
  Product_189a5/1 -> Product_f23a1/1
  Product_6f7df/1 -> Product_8548d/1
  Constant_f0_77ad9/1 -> Product_8548d/2
  Product_5c963/1 -> Product_6b28e/1
  Constant_f0_33950/1 -> Product_6b28e/2
  Divide_9ee5b/1 -> Add_c23fb/2
  Product_f23a1/1 -> Add_35dec/1
  Product_8548d/1 -> Add_35dec/2
  Product_6b28e/1 -> Product_4823a/1
  Add_c23fb/1 -> Product_4823a/2
  Add_35dec/1 -> Subtract_3e879/1
  Product_4823a/1 -> Subtract_3e879/2
  Constant_2.0_9f83b/1 -> Product_3826e/1
  Constant_H_8a38f/1 -> Product_3826e/2
  Subtract_3e879/1 -> Divide_f8d4a/1
  Product_3826e/1 -> Divide_f8d4a/2
  Divide_f8d4a/1 -> Blockout_d_w_SG_D_1_ca62c/1

== system case7/SG_D_1/i_d_SG_D_1_block ==
  note: i_d_SG_D_1 in case7
      | $\frac{\sin\left(\theta _{\mathrm{SG},D,1}\right)\,\left(\frac{\psi _{\mathrm{1d},\mathrm{SG},D,1}\,\left(x_{\mathrm{dd}}-x_{\mathrm{ddd}}\right)}{x_{\mathrm{dd}}-x_{l}}-\psi _{d,\mathrm{SG},D,1}+\frac{\psi _{\mathrm{fd},\mathrm{SG},D,1}\,\left(x_{\mathrm{ddd}}-x_{l}\right)}{x_{\mathrm{dd}}-x_{l}}\right)}{x_{\mathrm{ddd}}}-\frac{\cos\left(\theta _{\mathrm{SG},D,1}\right)\,\left(\psi _{q,\mathrm{SG},D,1}+\frac{\psi _{\mathrm{gq},\mathrm{SG},D,1}\,\left(x_{l}-x_{\mathrm{qdd}}\right)}{x_{l}-x_{\mathrm{qd}}}+\frac{\psi _{\mathrm{kq},\mathrm{SG},D,1}\,\left(x_{\mathrm{qd}}-x_{\mathrm{qdd}}\right)}{x_{l}-x_{\mathrm{qd}}}\right)}{x_{\mathrm{qdd}}}$
      | Automatically generated on 2025-10-31 19:23:52 .
  State_psi_gq_SG_D_1_613ce : Inport
  State_psi_kq_SG_D_1_5de85 : Inport  Port=2
  State_psi_q_SG_D_1_bff72 : Inport  Port=3
  State_theta_SG_D_1_6929e : Inport  Port=4
  State_psi_1d_SG_D_1_bfd03 : Inport  Port=5
  State_psi_d_SG_D_1_04ecd : Inport  Port=6
  State_psi_fd_SG_D_1_7462f : Inport  Port=7
  State_theta_SG_D_1_df07b : Inport  Port=8
  Add_5ced1 : Sum
  Add_63f38 : Sum
  Add_785a1 : Sum
  Add_aa7f4 : Sum
  Add_f8762 : Sum
  Constant_-1_40ff9 : Constant  Value=-1
  Constant_-1_4925d : Constant  Value=-1
  Constant_-1_60843 : Constant  Value=-1
  Constant_-1_c0aef : Constant  Value=-1
  Constant_-1_d22b5 : Constant  Value=-1
  Constant_x_dd_2ae2b : Constant  Value=x_dd
  Constant_x_dd_5d7a8 : Constant  Value=x_dd
  Constant_x_dd_9c281 : Constant  Value=x_dd
  Constant_x_ddd_39b7b : Constant  Value=x_ddd
  Constant_x_ddd_b1049 : Constant  Value=x_ddd
  Constant_x_ddd_d36a5 : Constant  Value=x_ddd
  Constant_x_l_2f880 : Constant  Value=x_l
  Constant_x_l_7f47c : Constant  Value=x_l
  Constant_x_l_9721a : Constant  Value=x_l
  Constant_x_l_9d254 : Constant  Value=x_l
  Constant_x_l_cc9c1 : Constant  Value=x_l
  Constant_x_l_eb631 : Constant  Value=x_l
  Constant_x_qd_1f196 : Constant  Value=x_qd
  Constant_x_qd_31192 : Constant  Value=x_qd
  Constant_x_qd_45413 : Constant  Value=x_qd
  Constant_x_qdd_085bc : Constant  Value=x_qdd
  Constant_x_qdd_75f33 : Constant  Value=x_qdd
  Constant_x_qdd_a2c04 : Constant  Value=x_qdd
  Divide_399f8 : Product  Inputs=*/
  Divide_aeafc : Product  Inputs=*/
  Divide_c419c : Product  Inputs=*/
  Divide_cdd2f : Product  Inputs=*/
  Divide_f1396 : Product  Inputs=*/
  Divide_feb9f : Product  Inputs=*/
  MathFunc_cos_28985 : Trigonometry  Operator=cos
  MathFunc_sin_1a492 : Trigonometry
  Product_100b7 : Product
  Product_240a4 : Product
  Product_248f0 : Product
  Product_2c602 : Product
  Product_305dc : Product
  Product_597c0 : Product
  Product_60f56 : Product
  Product_87379 : Product
  Product_a225c : Product
  Product_bb16e : Product
  Product_e4b0f : Product
  Subtract_16469 : Sum  Inputs=+-
  Subtract_2cb94 : Sum  Inputs=+-
  Subtract_31547 : Sum  Inputs=+-
  Subtract_593cc : Sum  Inputs=+-
  Subtract_5bcb3 : Sum  Inputs=+-
  Subtract_7708d : Sum  Inputs=+-
  Subtract_bc44d : Sum  Inputs=+-
  Subtract_f1429 : Sum  Inputs=+-
  Blockout_i_d_SG_D_1_6a835 : Outport
  wires:
  Constant_-1_4925d/1 -> Product_100b7/1
  Constant_x_l_9d254/1 -> Product_100b7/2
  Constant_x_ddd_39b7b/1 -> Subtract_593cc/2
  Product_100b7/1 -> Add_63f38/1
  Constant_x_qdd_75f33/1 -> Subtract_31547/2
  Constant_x_l_eb631/1 -> Product_305dc/2
  Constant_x_qd_31192/1 -> Add_5ced1/2
  Constant_x_qdd_a2c04/1 -> Add_63f38/2
  Constant_x_qd_1f196/1 -> Subtract_31547/1
  MathFunc_cos_28985/1 -> Product_87379/2
  Constant_-1_40ff9/1 -> Product_305dc/1
  Constant_-1_60843/1 -> Product_240a4/1
  Subtract_7708d/1 -> Blockout_i_d_SG_D_1_6a835/1
  Constant_x_l_cc9c1/1 -> Product_240a4/2
  Divide_cdd2f/1 -> Subtract_5bcb3/1
  State_psi_gq_SG_D_1_613ce/1 -> Product_2c602/1
  Subtract_2cb94/1 -> Product_60f56/2
  Add_63f38/1 -> Product_2c602/2
  Divide_feb9f/1 -> Add_785a1/1
  Product_305dc/1 -> Add_f8762/1
  Constant_x_qd_45413/1 -> Add_f8762/2
  State_psi_kq_SG_D_1_5de85/1 -> Product_a225c/1
  Add_785a1/1 -> Subtract_f1429/1
  Add_f8762/1 -> Divide_cdd2f/2
  Subtract_31547/1 -> Product_a225c/2
  Product_240a4/1 -> Add_5ced1/1
  Constant_-1_d22b5/1 -> Product_bb16e/1
  State_psi_1d_SG_D_1_bfd03/1 -> Product_bb16e/2
  Constant_x_dd_5d7a8/1 -> Subtract_593cc/1
  Product_2c602/1 -> Divide_cdd2f/1
  Product_248f0/1 -> Divide_399f8/1
  Subtract_593cc/1 -> Product_597c0/2
  Product_a225c/1 -> Divide_c419c/1
  Product_bb16e/1 -> Product_597c0/1
  Add_5ced1/1 -> Divide_c419c/2
  Constant_x_dd_2ae2b/1 -> Subtract_16469/1
  Subtract_5bcb3/1 -> Add_aa7f4/1
  Constant_x_l_7f47c/1 -> Subtract_16469/2
  Constant_x_ddd_b1049/1 -> Subtract_2cb94/1
  Constant_x_l_2f880/1 -> Subtract_2cb94/2
  Divide_399f8/1 -> Subtract_7708d/2
  Divide_c419c/1 -> Subtract_5bcb3/2
  State_theta_SG_D_1_6929e/1 -> MathFunc_cos_28985/1
  Product_597c0/1 -> Divide_feb9f/1
  Subtract_16469/1 -> Divide_feb9f/2
  State_theta_SG_D_1_df07b/1 -> MathFunc_sin_1a492/1
  State_psi_fd_SG_D_1_7462f/1 -> Product_60f56/1
  Constant_x_dd_9c281/1 -> Subtract_bc44d/1
  Constant_x_l_9721a/1 -> Subtract_bc44d/2
  State_psi_q_SG_D_1_bff72/1 -> Add_aa7f4/2
  State_psi_d_SG_D_1_04ecd/1 -> Add_785a1/2
  Constant_x_ddd_d36a5/1 -> Divide_399f8/2
  MathFunc_sin_1a492/1 -> Product_248f0/2
  Product_60f56/1 -> Divide_aeafc/1
  Constant_-1_c0aef/1 -> Product_e4b0f/1
  Subtract_bc44d/1 -> Divide_aeafc/2
  Add_aa7f4/1 -> Product_e4b0f/2
  Divide_aeafc/1 -> Subtract_f1429/2
  Product_e4b0f/1 -> Product_87379/1
  Subtract_f1429/1 -> Product_248f0/1
  Constant_x_qdd_085bc/1 -> Divide_f1396/2
  Product_87379/1 -> Divide_f1396/1
  Divide_f1396/1 -> Subtract_7708d/1

== system case7/SG_D_1/i_q_SG_D_1_block ==
  note: i_q_SG_D_1 in case7
      | $-\frac{\sin\left(\theta _{\mathrm{SG},D,1}\right)\,\left(\psi _{q,\mathrm{SG},D,1}+\frac{\psi _{\mathrm{gq},\mathrm{SG},D,1}\,\left(x_{l}-x_{\mathrm{qdd}}\right)}{x_{l}-x_{\mathrm{qd}}}+\frac{\psi _{\mathrm{kq},\mathrm{SG},D,1}\,\left(x_{\mathrm{qd}}-x_{\mathrm{qdd}}\right)}{x_{l}-x_{\mathrm{qd}}}\right)}{x_{\mathrm{qdd}}}-\frac{\cos\left(\theta _{\mathrm{SG},D,1}\right)\,\left(\frac{\psi _{\mathrm{1d},\mathrm{SG},D,1}\,\left(x_{\mathrm{dd}}-x_{\mathrm{ddd}}\right)}{x_{\mathrm{dd}}-x_{l}}-\psi _{d,\mathrm{SG},D,1}+\frac{\psi _{\mathrm{fd},\mathrm{SG},D,1}\,\left(x_{\mathrm{ddd}}-x_{l}\right)}{x_{\mathrm{dd}}-x_{l}}\right)}{x_{\mathrm{ddd}}}$
      | Automatically generated on 2025-10-31 19:23:54 .
  State_psi_gq_SG_D_1_d72fd : Inport
  State_psi_kq_SG_D_1_2e921 : Inport  Port=2
  State_psi_q_SG_D_1_25865 : Inport  Port=3
  State_theta_SG_D_1_37866 : Inport  Port=4
  State_psi_1d_SG_D_1_f3b13 : Inport  Port=5
  State_psi_d_SG_D_1_25480 : Inport  Port=6
  State_psi_fd_SG_D_1_21903 : Inport  Port=7
  State_theta_SG_D_1_2b1c8 : Inport  Port=8
  Add_0a9f9 : Sum
  Add_32b20 : Sum
  Add_554ca : Sum
  Add_8251c : Sum
  Add_abacd : Sum
  Add_f2473 : Sum
  Constant_-1_1bb55 : Constant  Value=-1
  Constant_-1_27430 : Constant  Value=-1
  Constant_-1_40472 : Constant  Value=-1
  Constant_-1_70e02 : Constant  Value=-1
  Constant_-1_88b47 : Constant  Value=-1
  Constant_x_dd_0d294 : Constant  Value=x_dd
  Constant_x_dd_9083d : Constant  Value=x_dd
  Constant_x_dd_dc7c4 : Constant  Value=x_dd
  Constant_x_ddd_87061 : Constant  Value=x_ddd
  Constant_x_ddd_893fc : Constant  Value=x_ddd
  Constant_x_ddd_90dbb : Constant  Value=x_ddd
  Constant_x_l_28834 : Constant  Value=x_l
  Constant_x_l_58fa2 : Constant  Value=x_l
  Constant_x_l_8c362 : Constant  Value=x_l
  Constant_x_l_ca377 : Constant  Value=x_l
  Constant_x_l_d1d71 : Constant  Value=x_l
  Constant_x_l_fc077 : Constant  Value=x_l
  Constant_x_qd_00beb : Constant  Value=x_qd
  Constant_x_qd_2d27c : Constant  Value=x_qd
  Constant_x_qd_59475 : Constant  Value=x_qd
  Constant_x_qdd_60db4 : Constant  Value=x_qdd
  Constant_x_qdd_a6e6f : Constant  Value=x_qdd
  Constant_x_qdd_bf45e : Constant  Value=x_qdd
  Divide_0972f : Product  Inputs=*/
  Divide_3ad68 : Product  Inputs=*/
  Divide_4d3f9 : Product  Inputs=*/
  Divide_5d68a : Product  Inputs=*/
  Divide_bcd17 : Product  Inputs=*/
  Divide_d8179 : Product  Inputs=*/
  MathFunc_cos_d7e3a : Trigonometry  Operator=cos
  MathFunc_sin_a85ea : Trigonometry
  Product_06f66 : Product
  Product_3a294 : Product
  Product_7eabd : Product
  Product_8d3c3 : Product
  Product_99f5d : Product
  Product_b2667 : Product
  Product_b69b7 : Product
  Product_c5999 : Product
  Product_e3c0d : Product
  Product_e43a2 : Product
  Product_f9a43 : Product
  Subtract_0497a : Sum  Inputs=+-
  Subtract_0bf0e : Sum  Inputs=+-
  Subtract_13a21 : Sum  Inputs=+-
  Subtract_7d5b8 : Sum  Inputs=+-
  Subtract_9dec6 : Sum  Inputs=+-
  Subtract_cf559 : Sum  Inputs=+-
  Subtract_e97bb : Sum  Inputs=+-
  Blockout_i_q_SG_D_1_6d7e3 : Outport
  wires:
  State_theta_SG_D_1_2b1c8/1 -> MathFunc_cos_d7e3a/1
  State_psi_fd_SG_D_1_21903/1 -> Product_8d3c3/1
  Constant_-1_88b47/1 -> Product_c5999/1
  Constant_x_l_ca377/1 -> Product_c5999/2
  Subtract_0bf0e/1 -> Product_8d3c3/2
  Constant_x_l_58fa2/1 -> Subtract_e97bb/2
  Product_c5999/1 -> Add_f2473/1
  Constant_x_qdd_bf45e/1 -> Add_f2473/2
  Constant_x_qd_2d27c/1 -> Subtract_7d5b8/1
  Constant_x_qdd_a6e6f/1 -> Divide_5d68a/2
  MathFunc_sin_a85ea/1 -> Product_b2667/2
  Constant_-1_27430/1 -> Product_3a294/1
  Constant_x_qdd_60db4/1 -> Subtract_7d5b8/2
  Add_abacd/1 -> Product_b69b7/2
  Product_e3c0d/1 -> Divide_4d3f9/1
  Constant_x_l_28834/1 -> Product_3a294/2
  Constant_-1_70e02/1 -> Product_99f5d/1
  Constant_x_l_d1d71/1 -> Product_99f5d/2
  State_psi_gq_SG_D_1_d72fd/1 -> Product_e3c0d/1
  Add_f2473/1 -> Product_e3c0d/2
  Divide_bcd17/1 -> Add_554ca/1
  Product_3a294/1 -> Add_8251c/1
  Divide_5d68a/1 -> Add_32b20/1
  Constant_x_qd_00beb/1 -> Add_8251c/2
  State_psi_kq_SG_D_1_2e921/1 -> Product_7eabd/1
  Add_554ca/1 -> Subtract_0497a/1
  Subtract_7d5b8/1 -> Product_7eabd/2
  Divide_4d3f9/1 -> Subtract_cf559/1
  Add_8251c/1 -> Divide_4d3f9/2
  Product_99f5d/1 -> Add_0a9f9/1
  Constant_x_qd_59475/1 -> Add_0a9f9/2
  Constant_-1_40472/1 -> Product_e43a2/1
  MathFunc_cos_d7e3a/1 -> Product_f9a43/2
  Product_8d3c3/1 -> Divide_0972f/1
  State_psi_1d_SG_D_1_f3b13/1 -> Product_e43a2/2
  Constant_x_l_fc077/1 -> Subtract_13a21/2
  Constant_x_dd_9083d/1 -> Subtract_9dec6/1
  Divide_0972f/1 -> Subtract_0497a/2
  Constant_x_ddd_90dbb/1 -> Subtract_9dec6/2
  Product_f9a43/1 -> Divide_d8179/1
  Product_7eabd/1 -> Divide_3ad68/1
  Product_e43a2/1 -> Product_06f66/1
  Add_0a9f9/1 -> Divide_3ad68/2
  Subtract_9dec6/1 -> Product_06f66/2
  State_psi_d_SG_D_1_25480/1 -> Add_554ca/2
  Constant_x_dd_dc7c4/1 -> Subtract_e97bb/1
  Constant_x_ddd_893fc/1 -> Subtract_0bf0e/1
  Constant_x_l_8c362/1 -> Subtract_0bf0e/2
  Divide_d8179/1 -> Add_32b20/2
  Divide_3ad68/1 -> Subtract_cf559/2
  State_theta_SG_D_1_37866/1 -> MathFunc_sin_a85ea/1
  Product_06f66/1 -> Divide_bcd17/1
  Subtract_e97bb/1 -> Divide_bcd17/2
  Constant_x_dd_0d294/1 -> Subtract_13a21/1
  Subtract_cf559/1 -> Add_abacd/1
  State_psi_q_SG_D_1_25865/1 -> Add_abacd/2
  Subtract_13a21/1 -> Divide_0972f/2
  Subtract_0497a/1 -> Product_f9a43/1
  Constant_-1_1bb55/1 -> Product_b69b7/1
  Product_b69b7/1 -> Product_b2667/1
  Product_b2667/1 -> Divide_5d68a/1
  Constant_x_ddd_87061/1 -> Divide_d8179/2
  Add_32b20/1 -> Blockout_i_q_SG_D_1_6d7e3/1

== system case7/SG_D_1/theta_SG_D_1_out_block ==
  note: theta_SG_D_1_out in case7
      | $\theta _{\mathrm{SG},D,1}$
      | Automatically generated on 2025-10-31 19:23:59 .
  State_theta_SG_D_1_a05eb : Inport
  Blockout_theta_SG_D_1_out_771f4 : Outport
  wires:
  State_theta_SG_D_1_a05eb/1 -> Blockout_theta_SG_D_1_out_771f4/1

== system case7/SG_D_1/w_SG_D_1_out_block ==
  note: w_SG_D_1_out in case7
      | $w_{\mathrm{SG},D,1}$
      | Automatically generated on 2025-10-31 19:23:58 .
  State_w_SG_D_1_b6dd0 : Inport
  Blockout_w_SG_D_1_out_64aa4 : Outport
  wires:
  State_w_SG_D_1_b6dd0/1 -> Blockout_w_SG_D_1_out_64aa4/1
